simulink model "APB_Model0_v03_Test"  (R2020b)
settings: Solver=ode45  StartTime=0.0  StopTime=inf  RelTol=1e-3
undefined symbols (not defined in the file or in its folder): calb_Driver_acce, calb_Driver_bttn, calb_Driver_EmrBrk, calb_Driver_Prss, G_Fclamp, G_Kmot, G_Rmot, G_Stroke, G_SwOmega, GEN3, PbcDataStorageRequest_t
libraries: etargetslib x26, Lib_Op_Hndl x4, simulink x2, PbcOut_Checksum x2
(part 3 of 5)

== system APB_Model0_v03_Test/HstEcu/PBC/Subsystem/Subsystem3 ==
  PBCInMotorCurrentLeft_1ms : Inport
  Constant : Constant  Value=GEN3
  Delay : Delay  DelayLength=1
  Subsystem : Subsystem
  Subsystem4 : Subsystem
  Switch : Switch  Criteria=u2 ~= 0
  <phys_HwDrCt_ImotL> : Outport
  wires:
  Constant/1 -> Switch/2
  Subsystem4/1(Out1) -> Switch/1
  Subsystem/1(Out1) -> Switch/3
  Switch/1 -> <phys_HwDrCt_ImotL>/1
  PBCInMotorCurrentLeft_1ms/1 -> Delay/1
  Delay/1 -> Subsystem4/1(PBCInMotorCurrentLeft_1ms), Subsystem/1(PBCInMotorCurrentLeft_1ms)

== system APB_Model0_v03_Test/HstEcu/PBC/Subsystem/Subsystem4 ==
  PBCInMotorCurrentLeft_1ms : Inport
  Constant : Constant  Value=GEN3
  Delay : Delay  DelayLength=1
  Subsystem : Subsystem
  Subsystem4 : Subsystem
  Switch : Switch  Criteria=u2 ~= 0
  <phys_HwDrCt_ImotL> : Outport
  wires:
  PBCInMotorCurrentLeft_1ms/1 -> Delay/1
  Switch/1 -> <phys_HwDrCt_ImotL>/1
  Subsystem/1(Out1) -> Switch/3
  Subsystem4/1(Out1) -> Switch/1
  Constant/1 -> Switch/2
  Delay/1 -> Subsystem/1(PBCInMotorCurrentLeft_1ms), Subsystem4/1(PBCInMotorCurrentLeft_1ms)

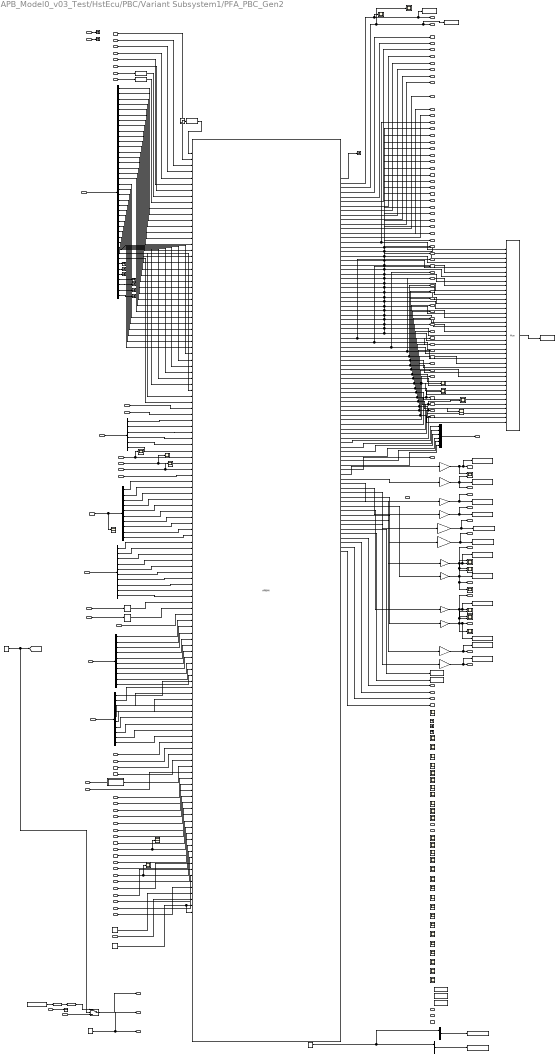
== system APB_Model0_v03_Test/HstEcu/PBC/Variant Subsystem1/PFA_PBC_Gen2 ==
  Pbc_Init : Inport
  Pbc_Cyclic : Inport  Port=2
  ApplyReleaseRequest : Inport  Port=3
  PBCInRollerBenchActive : Inport  Port=4
  PBCInLongAcceleration : Inport  Port=5
  PBCInMasterCylinderPressure : Inport  Port=6
  PBCInVehicleAmbientTemperature : Inport  Port=7
  PBCInWheelPressureFL : Inport  Port=8
  PBCInWheelPressureFR : Inport  Port=9
  PBCInWheelPressureRL : Inport  Port=10
  PBCInWheelPressureRR : Inport  Port=11
  PBCInWheelPressureReliabilityFL : Inport  Port=12
  PBCInWheelPressureReliabilityFR : Inport  Port=13
  PBCInWheelPressureReliabilityRL : Inport  Port=14
  PBCInWheelPressureReliabilityRR : Inport  Port=15
  PBCInWheelPulseFL : Inport  Port=16
  PBCInWheelPulseFR : Inport  Port=17
  PBCInWheelPulseRL : Inport  Port=18
  PBCInWheelPulseRR : Inport  Port=19
  PBCInWheelSPeedFL : Inport  Port=20
  PBCInWheelSPeedFR : Inport  Port=21
  PBCInWheelSPeedRL : Inport  Port=22
  PBCInWheelSPeedRR : Inport  Port=23
  PBCInDiagOperationMode : Inport  Port=24
  PBCInDiagRequest : Inport  Port=25
  PBCinHostSoftwareVersion : Inport  Port=26
  PBCInDataStorageValid1 : Inport  Port=27
  PBCInDataStorageValid2 : Inport  Port=28
  PBCInDataStorageValid3 : Inport  Port=29
  PBCInUnexpectedPowerDown : Inport  Port=30
  PBCInVariantItem : Inport  Port=31
  PBCInDataStorageRead1 : Inport  Port=32
  PBCInDataStorageRead9 : Inport  Port=33
  PBCInPbcSleepTime : Inport  Port=34
  PBCInFaultRecoveryRequest : Inport  Port=35
  PBCInHpsAvailability : Inport  Port=36
  PBCInHpsAcknowledge : Inport  Port=37
  PBCInMotorCurrentLeft_1ms : Inport  Port=38
  PBCInMotorCurrentRight_1ms : Inport  Port=39
  HWDriver_MotorVoltageLeft_1ms : Inport  Port=40
  HWDriver_MotorVoltageRight_1ms : Inport  Port=41
  PBCInMotorDriverSupplyVoltage : Inport  Port=42
  PBCinHostAvailabilityLeft : Inport  Port=43
  PBCinHostAvailabilityRight : Inport  Port=44
  PBCInMotorDriverStateLeft : Inport  Port=45
  PBCInMotorDriverStateRight : Inport  Port=46
  PBCInPowerSupplyState : Inport  Port=47
  PbcInMileage : Inport  Port=48
  PbcInEngineCranking : Inport  Port=49
  PbcInDriveAwayIntentionIndication : Inport  Port=50
  "PBCInDataStorageRead77 " : Inport  Port=51
  "PBCInDataStorage_Read " : Inport  Port=52
  OutOfSpec_Init : Inport  Port=53
  AcP00 : Scope
  AcP77 : Scope
  AcpData02 : Scope
  AcpData04 : Scope
  AssemblyChek : Scope
  Constant : Constant  Value=0
  Constant1 : Constant  Value=0
  Constant2 : Constant  Value=0  OutDataTypeStr=uint8
  Constant4 : Constant  Value=0
  Constant9 : Constant  Value=0  OutDataTypeStr=uint8
  Data Type Conversion{1,5,7..8} (4 alike) : DataTypeConversion  OutDataTypeStr=uint8
  Data Type Conversion6 : DataTypeConversion  OutDataTypeStr=boolean
  Data03 : Scope
  Data255 : Scope
  Demux1 : Demux  Outputs=40
  Demux{2..5} (4 alike) : Demux  Outputs=10
  Demux6 : Demux  Outputs=6
  EncodedAssembly : Scope
  From Workspace : FromWorkspace  VariableName=Memo1
  Gain{1,8,11..12} (4 alike) : Gain  Gain=G_Fclamp
  Gain10 : Gain  Gain=G_Rmot
  Gain2 : Gain  Gain=G_Stroke
  Gain3 : Gain  Gain=G_Stroke
  Gain4 : Gain  Gain=G_SwOmega
  Gain5 : Gain  Gain=G_SwOmega
  Gain6 : Gain  Gain=G_Kmot
  Gain7 : Gain  Gain=G_Kmot
  Gain9 : Gain  Gain=G_Rmot
  IsAllData : Scope
  IsAllDataInit : Scope
  IsIf1Reached : Scope
  IsIfaActive : Scope
  IsRelfinis : Scope  NumInputPorts=2
  Mux : Mux  Inputs=2
  Mux1 : Mux  Inputs=2
  Mux2 : Mux  Inputs=6
  Mux3 : Mux  Inputs=5
  Mux4 : Mux  Inputs=39
  Rate Transition42 : RateTransition  OutPortSampleTime=0.01
      settings: AttributesFormatString=%<OutPortSampleTime>
  Rate Transition43 : RateTransition  OutPortSampleTime=0.01
      settings: AttributesFormatString=%<OutPortSampleTime>
  ReleaseTim : Scope  NumInputPorts=2
  S-Function Builder1 : S-Function  InitFcn=try, set_param(gcb,'FunctionName','APBMi'), end  FunctionName=APBMi  SFunctionModules=APBMi_wrapper AcmBtmCalcStartBit AcmBtmCoolingAdjustmentConditions AcmBtmDTDiscCalcCooling AcmBtmDTDiscCalcHeating AcmBtmDTDiscSum AcmBtmFailureConditions AcmBtmInitStandstillCorrection AcmBtmMain AcmBtmOverheatCalc AcmBtmQualifierUpgrade AcmBtmSetFaultHandler AcmBtmSigPerm AcmBtmStatusCoding AcmBtmTambUpdate AcmBtmTDisc AcmBtmTrigger AcmBtmVelocityUpdate AcmBtmWheelXY AcpHemming AcpLibInCopy AcpLibOutCopy AcpLibWrapper AcpVariant ActuateReclamp ApplyPhaseStateMachine Ax2SlopeRaw a_intpol BtmInterfaceAdaption BtmTaskAdaption calcPbcActualMotorCommand calcPbcTargetMotorCommand CalcPostRunReq calcSwOmegaDot calcTargetStateDA Cal_VehicleSpeed ChangeTypeOfRC_HpsNotAcknowledged ChangeTypeOfRC_RDF_WithoutHps ChoiceOfCFS confEcuCodeGen_VDA_2 DataResetRequestDistinction Decoder_WSS_Quality DelayTimeCalculation DiagExecutionHandler DiagModeFConnectorOut DiagReqFeedback DiagRequestAccepter DiagRequestAckowledge_Enum_Map DiagRequestSplitter DiagRequest_Enum_Map DiagStateCalculation DiagStateHandler DSM_EmergencyReleaseSwitch DSM_FailureNode DSM_HostAvailabilityDecoder DSM_MainFailureHandler DSM_TargetStateIndependant DSM_TargetStateMain DSM_TargetStateMax dx_dt dx_dt0 EEPROM_Decoder_C EEPROM_Encoder_C EngineCranking ErrorRatioGoodCheckEncoder ForceEstimation HFBA_Repeater HostAvailabilityDetection HpsActivator HpsMerging HpsPressureChoice HpsSteering IfaTif_StateMachine InfoAchievedFClamp InfoAppCounter InfoBrakeTemperature InfoFLOne_TwoCounter InfoHPSRequestCounter InfoOutOfSpec InfoReclampCounter InfoReleaseCounter InitialConditionsforRWU InitStateCalculation isEndOfIdlePhase isForceEstimationActivate isMotParValid isRwuExecutionPossible isSwitchOnPeakPresent isTDiscRearMaxValid LateEngineCranking LockReleaseExecutionHandler LockReleaseStatemachine MileageSinceLastParkApplied MileageValidity MocOff_DeltaF_Addition MonIDs MON_ActuatorModeInitMonitoring MON_ActuatorModeOperationMonitoring MON_DegradationManager MON_DevEncoder MON_DevEncoderInit_APBDi MON_DiagnosisDetector MON_DynLockDetector MON_EmergencyReleaseDetectionDurRel MON_EngineCranking MON_ErrorRatioGoodCheckEncoder MON_GradientMonitoringForceBuildUpDurLock MON_HPSRequestFailureDurLock MON_IdleSpindleStrokeMonitoringDurLock MON_IdleTorqueMonitoringDurLock MON_MotorControlDetectionDurAppl MON_MotorParameterMonitoringDurLock MON_TimeoutMonitoringForceBuildUpDurLock NoActuation OngoingActuation OnGoingActuationExtended OutOfSpec PAAMerging PadAdjustmentRequest ParAcp_BrakeDiscTemperatureModel ParAcp_BTM_Calibration ParAcp_BTM_FA ParAcp_BTM_RA ParAcp_Constant ParAcp_DynamicStateManager ParAcp_HpsDevice ParAcp_HWDriver ParAcp_InfoService ParAcp_Monitoring ParAcp_MotorControl ParAcp_PadAdjust ParAcp_RecalibrationFunction ParAcp_RollDetection ParAcp_RWU ParAcp_SlopeCalculation ParAcp_TargetActuation ParkBrakeControl_T10ms_VDA_2 ParkBrakeControl_VDA_2 PbcBTM PbcBTM_PdmValueValidAdaption PbcChronometre PbcCtrlBothWheels PbcCtrlOneWheel PbcDynamicStateManager PbcForceEstimation PbcHpsChronometre PbcHpsDevice PbcHWDriverCommand PbcHWDriverCommandBothWheels PbcIfPDM PbcInfoService PbcMotorControl PbcMovementDetection PbcPadAdjustment PbcQDotReader PbcQDotReaderSoPeak PbcRecalibrationFunction PbcRoadSlope_availability PbcRollDetection PbcRWU PbcRwuSlip PbcSignalConditioning PbcSlopeCalculation PbcSpeedCalculation PbcTargetActuation PbcVehicleMovementDetection PbcWheelMovementDetection PBC_BoschCbi_VDA_2 Pbc_dcTLA Pbc_dcTLA_ClampingForceTable Pbc_DcTLA_StateMachine Pbc_FClampTarBySlope_CBI Pbc_ParkBrakeSupportRequest Pbc_prepressure_calculation Pbc_Pressure4StandstillDetection_CBI Pbc_ReclampType_Merging Pbc_VDAtwo Pbc_VHC PdmActuatorState PdmBtm PdmDataValid PTAMerging RecalibrationTrigger RecogTouchPoints RollAwayValidation RollerBenchHandler RWU_StateMachine SIC_APBMi SIC_Calc_R_K_Mot SIC_IdlePhaseParameter SIC_InrushPeakDetector SIC_MotorCurrent SIC_MotorCurrentConcentrator SIC_MotorCurrentCtrl SIC_MotorParameter SIC_MotorResidualCurrent SIC_MotorVoltage SIC_PistonStroke Signal_Availability_sint Signal_Availability_sint0 Signal_Availability_sint1 Signal_Availability_uint Signal_Availability_uint0 Signal_Availability_uint1 StateRequestCalculation StopImmediatelyCalculation StopImmediatelyCalculationLR TargetStateRDF TestCalc0xFF TestValue_C WheelPressureReliability_Enum_Map _BTM_Constant _Environment_QualityGrades MON_APBMi ActuateAllReleases ActuateByForce ActuatorStateMerging ApplyReleaseMerging CFS_IndependentActuation DevelopmentMessagesEncoding DevelpmentMessagesPreparation DiagModeFConnector DoubleApplyFunction DSM_FaultStatusMerging EEPROM_Boolean_Coder ForceEstimationVoltTempFactor HpsRequestMerging IndependantActuationConfig InfoOutOfSpecBlock isActuatorFinalState LongAccelerationManagement MergeParkBrakeSupportRequest MON_AbutmentDetectionDurRel MON_DisableMonitoring MON_ForcedGoodCheck MON_FreeLoadDetectionDurRel MON_HostDown MON_InfoFaultMonitoring MON_LeftRightIncoherence MON_MotorStartDetection MON_Overvoltage MON_SideSelfIncoherence MON_SuspicousReleasedDetector MON_Undervoltage OosActivator OosAxInvalid OosCbiStar OosDataStorage3Invalid OosIndependentControl OosMerger OosSlopeInvalid ParAcp_ForceEstimation ParAcp_InputHandling ParAcp_SignalConditioning Pbc_FClamp_PostRunTimeTgt Pbc_hRCWithoutHps Pbc_TemperatureSlopePressure_SliceChoice PbcDevelopmentMessages PbcForceEstimationOp PbcInputHandler PbcPistonPositionEstimation PbcVariantConfig PdmRollAway RequestProcesser TestCalcInit WaitRecoveryActuationEnded HostAvailabilityMerging Pbc_ReleaseStroke_Calculation VoltageVariationDetection  SFunctionDeploymentMode=off  EnableBusSupport=off  mask(S-Function Builder){}
      mask help: The S-Function Builder block creates a wrapper C-MEX S-function from your supplied C code with multiple input ports, output ports, and a variable number of scalar, vector, or matrix parameters. The input and output ports can propagate Simulink built-in data types, fixed-point datatypes, complex, frame, 1-D, and 2-D signals. This block also supports discrete and continuous states of type real. You can optionally have the block generate a TLC file to be used with Real-Time Workshop for code generation.
      mask init:
      | val = [[.9  0.75 0.75 1 1 .9 .9 1]',[1 1 0.75 0.75 .9 .9 1 .9]'];try , sys = get_param(gcb,'SfunBuilderFcnName');if isempty(sys), sys = get_param(gcb,'FunctionName'); end,catch, sys = get_param(gcb,'FunctionName'); end
      settings: AttributesFormatString=%<SFunctionModules>\n%<FunctionName>  CopyFcn=set_param(gcbh,'LinkStatus','none')  PreSaveFcn=try, set_param(gcb,'FunctionName','APBMi'), end  OpenFcn=sfunctionwizard(gcbh)
      mask Display: plot(val(:,1),val(:,2)),disp(sys),port_label('input',1,'triggerInFirstCall'),port_label('input',2,'PBCInApplyReleaseRequest'),port_label('input',3,'PBCInDataStorageRead1'),port_label('input',4,'PBCInDataStorageRead9'),port_label('input',5,'PBCInDataStorageValid1'),port_label('input',6,'PBCInDataStorageValid2'),port_label('input',7,'PBCInDataStorageValid3'),port_label('input',8,'PBCInDiagOperationMode'),port_label('input',9,'PBCInDiagRequest'),port_label('input',10,'PBCInFaultRecoveryRequest_01'),port_label('input',11,'PBCInFaultRecoveryRequest_02'),port_label('input',12,'PBCInFaultRecoveryRequest_03'),port_label('input',13,'PBCInFaultRecoveryRequest_04'),port_label('input',14,'PBCInFaultRecoveryRequest_05'),port_label('input',15,'PBCInFaultRecoveryRequest_06'),port_label('input',16,'PBCInFaultRecoveryRequest_07'),port_label('input',17,'PBCInFaultRecoveryRequest_08'),port_label('input',18,'PBCInFaultRecoveryRequest_09'),port_label('input',19,'PBCInFaultRecoveryRequest_10'),port_label('input',20,'PBCInFaultRecoveryRequest_11'),port_label('input',21,'PBCInFaultRecoveryRequest_12'),port_label('input',22,'PBCInFaultRecoveryRequest_13'),port_label('input',23,'PBCInFaultRecoveryRequest_14'),port_label('input',24,'PBCInFaultRecoveryRequest_15'),port_label('input',25,'PBCInFaultRecoveryRequest_16'),port_label('input',26,'PBCInFaultRecoveryRequest_17'),port_label('input',27,'PBCInFaultRecoveryRequest_18'),port_label('input',28,'PBCInFaultRecoveryRequest_19'),port_label('input',29,'PBCInFaultRecoveryRequest_20'),port_label('input',30,'PBCInFaultRecoveryRequest_21'),port_label('input',31,'PBCInFaultRecoveryRequest_22'),port_label('input',32,'PBCInFaultRecoveryRequest_23'),port_label('input',33,'PBCInFaultRecoveryRequest_24'),port_label('input',34,'PBCInFaultRecoveryRequest_25'),port_label('input',35,'PBCInFaultRecoveryRequest_26'),port_label('input',36,'PBCInFaultRecoveryRequest_27'),port_label('input',37,'PBCInFaultRecoveryRequest_29'),port_label('input',38,'PBCInFaultRecoveryRequest_30'),port_label('input',39,'PBCInFaultRecoveryRequest_31'),port_label('input',40,'PBCInFaultRecoveryRequest_32'),port_label('input',41,'PBCInFaultRecoveryRequest_33'),port_label('input',42,'PBCInFaultRecoveryRequest_39'),port_label('input',43,'PBCInHostAvailabilityLeft'),port_label('input',44,'PBCInHostAvailabilityRight'),port_label('input',45,'PBCInHostSoftwareVersion0'),port_label('input',46,'PBCInHostSoftwareVersion1'),port_label('input',47,'PBCInHostSoftwareVersion2'),port_label('input',48,'PBCInHostSoftwareVersion3'),port_label('input',49,'PBCInHostSoftwareVersion4'),port_label('input',50,'PBCInHostSoftwareVersion5'),port_label('input',51,'PBCInHpsAvailability'),port_label('input',52,'PBCInHpsAcknowledge'),port_label('input',53,'PBCInLongAcceleration'),port_label('input',54,'PBCInMasterCylinderPressure'),port_label('input',55,'PBCInMotorCurrentLeft_K0'),port_label('input',56,'PBCInMotorCurrentLeft_K1'),port_label('input',57,'PBCInMotorCurrentLeft_K2'),port_label('input',58,'PBCInMotorCurrentLeft_K3'),port_label('input',59,'PBCInMotorCurrentLeft_K4'),port_label('input',60,'PBCInMotorCurrentLeft_K5'),port_label('input',61,'PBCInMotorCurrentLeft_K6'),port_label('input',62,'PBCInMotorCurrentLeft_K7'),port_label('input',63,'PBCInMotorCurrentLeft_K8'),port_label('input',64,'PBCInMotorCurrentLeft_K9'),port_label('input',65,'PBCInMotorCurrentRight_K0'),port_label('input',66,'PBCInMotorCurrentRight_K1'),port_label('input',67,'PBCInMotorCurrentRight_K2'),port_label('input',68,'PBCInMotorCurrentRight_K3'),port_label('input',69,'PBCInMotorCurrentRight_K4'),port_label('input',70,'PBCInMotorCurrentRight_K5'),port_label('input',71,'PBCInMotorCurrentRight_K6'),port_label('input',72,'PBCInMotorCurrentRight_K7'),port_label('input',73,'PBCInMotorCurrentRight_K8'),port_label('input',74,'PBCInMotorCurrentRight_K9'),port_label('input',75,'PBCInMotorDriverStateLeft'),port_label('input',76,'PBCInMotorDriverStateRight'),port_label('input',77,'PBCInMotorDriverSupplyVoltage'),port_label('input',78,'PBCInMotorVoltageLeft_K0'),port_label('input',79,'PBCInMotorVoltageLeft_K1'),port_label('input',80,'PBCInMotorVoltageLeft_K2'),port_label('input',81,'PBCInMotorVoltageLeft_K3'),port_label('input',82,'PBCInMotorVoltageLeft_K4'),port_label('input',83,'PBCInMotorVoltageLeft_K5'),port_label('input',84,'PBCInMotorVoltageLeft_K6'),port_label('input',85,'PBCInMotorVoltageLeft_K7'),port_label('input',86,'PBCInMotorVoltageLeft_K8'),port_label('input',87,'PBCInMotorVoltageLeft_K9'),port_label('input',88,'PBCInMotorVoltageRight_K0'),port_label('input',89,'PBCInMotorVoltageRight_K1'),port_label('input',90,'PBCInMotorVoltageRight_K2'),port_label('input',91,'PBCInMotorVoltageRight_K3'),port_label('input',92,'PBCInMotorVoltageRight_K4'),port_label('input',93,'PBCInMotorVoltageRight_K5'),port_label('input',94,'PBCInMotorVoltageRight_K6'),port_label('input',95,'PBCInMotorVoltageRight_K7'),port_label('input',96,'PBCInMotorVoltageRight_K8'),port_label('input',97,'PBCInMotorVoltageRight_K9'),port_label('input',98,'PBCInPowerSupplyState'),port_label('input',99,'PBCInRollerBenchActive'),port_label('input',100,'PBCInPbcSleepTime'),port_label('input',101,'PBCInUnexpectedPowerDown'),port_label('input',102,'PBCInVariantItem'),port_label('input',103,'PBCInVehicleAmbientTemperature'),port_label('input',104,'PBCInWheelPressureFrontLeft'),port_label('input',105,'PBCInWheelPressureFrontRight'),port_label('input',106,'PBCInWheelPressureRearLeft'),port_label('input',107,'PBCInWheelPressureRearRight'),port_label('input',108,'PBCInWheelPressureReliabilityFrontLeft'),port_label('input',109,'PBCInWheelPressureReliabilityFrontRight'),port_label('input',110,'PBCInWheelPressureReliabilityRearLeft'),port_label('input',111,'PBCInWheelPressureReliabilityRearRight'),port_label('input',112,'PBCInWheelPulseFrontLeft'),port_label('input',113,'PBCInWheelPulseFrontRight'),port_label('input',114,'PBCInWheelPulseRearLeft'),port_label('input',115,'PBCInWheelPulseRearRight'),port_label('input',116,'PBCInWheelSpeedFrontLeft'),port_label('input',117,'PBCInWheelSpeedFrontRight'),port_label('input',118,'PBCInWheelSpeedRearLeft'),port_label('input',119,'PBCInWheelSpeedRearRight'),port_label('input',120,'PbcInEngineCranking'),port_label('input',121,'PbcInMileage'),port_label('input',122,'PbcInDriveAwayIntentionIndication'),port_label('input',123,'PBCInDataStorageRead105'),port_label('input',124,'PBCInDataStorageRead77'),port_label('input',125,'PBCInDataStorageRead80'),port_label('input',126,'PBCInDataStorageRead91'),port_label('input',127,'PBCInDataStorageRead92'),port_label('input',128,'PBCInDataStorageRead93'),port_label('input',129,'PBCInDataStorageRead94'),port_label('input',130,'PBCInDataStorageRead95'),port_label('input',131,'PBCInDataStorageRead96'),port_label('input',132,'PBCInDataStorageRead97'),port_label('input',133,'PBCInDataStorageRead2'),port_label('input',134,'PBCInDataStorageRead3'),port_label('input',135,'PBCInDataStorageRead10'),port_label('input',136,'PBCInDataStorageRead142'),port_label('input',137,'MDbgFClampTar'),port_label('input',138,'MDbg_factorV_Left_F1'),port_label('input',139,'MDbg_factorT_Left_F1'),port_label('input',140,'MDbg_factorV_Left_F2'),port_label('input',141,'MDbg_factorT_Left_F2'),port_label('input',142,'MDbg_factorV_Right_F1'),port_label('input',143,'MDbg_factorT_Right_F1'),port_label('input',144,'MDbg_factorV_Right_F2'),port_label('input',145,'MDbg_factorT_Right_F2'),port_label('output',1,'triggerOutFirstCall'),port_label('output',2,'PBCOutActuatorStateLeft'),port_label('output',3,'PBCOutActuatorStateRight'),port_label('output',4,'PBCOutDataStorageWrite1'),port_label('output',5,'PBCOutDataStorageWrite9'),port_label('output',6,'PBCOutDevelopmentMessages0'),port_label('output',7,'PBCOutDiagAchievedClampingForceLeft'),port_label('output',8,'PBCOutDiagAchievedClampingForceRight'),port_label('output',9,'PBCOutDiagActuationCounterLeft'),port_label('output',10,'PBCOutDiagActuationCounterRight'),port_label('output',11,'PBCOutDiagBrakeTemperatureLeft'),port_label('output',12,'PBCOutDiagBrakeTemperatureRight'),port_label('output',13,'PBCOutDiagRequestAcknowledge'),port_label('output',14,'PBCOutDiagRequestStatus'),port_label('output',15,'PBCOutFaultStatus_01'),port_label('output',16,'PBCOutFaultStatus_02'),port_label('output',17,'PBCOutFaultStatus_03'),port_label('output',18,'PBCOutFaultStatus_04'),port_label('output',19,'PBCOutFaultStatus_05'),port_label('output',20,'PBCOutFaultStatus_06'),port_label('output',21,'PBCOutFaultStatus_07'),port_label('output',22,'PBCOutFaultStatus_08'),port_label('output',23,'PBCOutFaultStatus_09'),port_label('output',24,'PBCOutFaultStatus_10'),port_label('output',25,'PBCOutFaultStatus_11'),port_label('output',26,'PBCOutFaultStatus_12'),port_label('output',27,'PBCOutFaultStatus_13'),port_label('output',28,'PBCOutFaultStatus_14'),port_label('output',29,'PBCOutFaultStatus_15'),port_label('output',30,'PBCOutFaultStatus_16'),port_label('output',31,'PBCOutFaultStatus_17'),port_label('output',32,'PBCOutFaultStatus_18'),port_label('output',33,'PBCOutFaultStatus_19'),port_label('output',34,'PBCOutFaultStatus_20'),port_label('output',35,'PBCOutFaultStatus_21'),port_label('output',36,'PBCOutFaultStatus_22'),port_label('output',37,'PBCOutFaultStatus_23'),port_label('output',38,'PBCOutFaultStatus_24'),port_label('output',39,'PBCOutFaultStatus_25'),port_label('output',40,'PBCOutFaultStatus_26'),port_label('output',41,'PBCOutFaultStatus_27'),port_label('output',42,'PBCOutFaultStatus_28'),port_label('output',43,'PBCOutFaultStatus_29'),port_label('output',44,'PBCOutFaultStatus_30'),port_label('output',45,'PBCOutFaultStatus_31'),port_label('output',46,'PBCOutFaultStatus_32'),port_label('output',47,'PBCOutFaultStatus_33'),port_label('output',48,'PBCOutFaultStatus_34'),port_label('output',49,'PBCOutFaultStatus_35'),port_label('output',50,'PBCOutFaultStatus_36'),port_label('output',51,'PBCOutFaultStatus_37'),port_label('output',52,'PBCOutFaultStatus_38'),port_label('output',53,'PBCOutFaultStatus_39'),port_label('output',54,'PBCOutHpsPressure'),port_label('output',55,'PBCOutHpsRequest'),port_label('output',56,'PBCOutMotorCommandLeft'),port_label('output',57,'PBCOutMotorCommandRight'),port_label('output',58,'PBCOutOutOfSpecMsg'),port_label('output',59,'PBCOutPbcSoftwareVersion0'),port_label('output',60,'PBCOutPbcSoftwareVersion1'),port_label('output',61,'PBCOutPbcSoftwareVersion2'),port_label('output',62,'PBCOutPbcSoftwareVersion3'),port_label('output',63,'PBCOutPbcSoftwareVersion4'),port_label('output',64,'PBCOutPbcSoftwareVersion5'),port_label('output',65,'PBCOutEcuPowerLatchRequest'),port_label('output',66,'PBCinternalFclampR'),port_label('output',67,'PBCinternalFclampL'),port_label('output',68,'PBCinternalSwStrokeR'),port_label('output',69,'PBCinternalSwStrokeL'),port_label('output',70,'PBCinternalSwOmegaR'),port_label('output',71,'PBCinternalSwOmegaL'),port_label('output',72,'PBCinternalKMotR'),port_label('output',73,'PBCinternalKMotL'),port_label('output',74,'PBCinternalRMotR'),port_label('output',75,'PBCinternalRMotL'),port_label('output',76,'PBCinternalFtarR'),port_label('output',77,'PBCinternalFtarL'),port_label('output',78,'PBCinternalTargetActuationR'),port_label('output',79,'PBCinternalTargetActuationL'),port_label('output',80,'PbcOutPadAdjustmentRequest'),port_label('output',81,'PbcOutParkSupportRequest'),port_label('output',82,'PbcOutDataStorageRequest'),port_label('output',83,'TriggerRecalibration'),port_label('output',84,'FachivedL'),port_label('output',85,'FachivedR'),port_label('output',86,'apprealreq'),port_label('output',87,'Motorcurrent'),port_label('output',88,'Motorvoltage'),port_label('output',89,'version4'),port_label('output',90,'version3'),port_label('output',91,'version2'),port_label('output',92,'version1'),port_label('output',93,'version0'),port_label('output',94,'MApplyReleaseRequestin'),port_label('output',95,'MTargetStateMainL'),port_label('output',96,'MTargetStateMainR'),port_label('output',97,'MUMotFLeft'),port_label('output',98,'MIMotFLeft'),port_label('output',99,'MIMotByForceLeft'),port_label('output',100,'MIMotResLeft'),port_label('output',101,'MIMotGradLeft'),port_label('output',102,'MIMotIdleLeft'),port_label('output',103,'MIMotIdleSeqLeft'),port_label('output',104,'MUMotIdleLeft'),port_label('output',105,'MKMotLeft'),port_label('output',106,'MRMotLeft'),port_label('output',107,'MMotParamQualifierLeft'),port_label('output',108,'MPistonStrokeLeft'),port_label('output',109,'MPistonStrokeFreeLoadLeft'),port_label('output',110,'MPistonStrokeFreeLoadT1Left'),port_label('output',111,'MPistonStrokeFreeLoadT2Left'),port_label('output',112,'MPistonStrokeT1Left'),port_label('output',113,'MPistonStrokeT2Left'),port_label('output',114,'MwMotFLeft'),port_label('output',115,'MPbcApplyPhaseLeft'),port_label('output',116,'MFEstLeft'),port_label('output',117,'MMInertiaLeft'),port_label('output',118,'MDeltaF_FEstLeft'),port_label('output',119,'MFEst_incl_MoCOffLeft'),port_label('output',120,'MFEstoptimalVTLeft'),port_label('output',121,'MisOuterAbutmentTouchedLeft'),port_label('output',122,'MisTouchPointReachedLeft'),port_label('output',123,'MPbcTargetMotorCommandLeft'),port_label('output',124,'MisActuationFinishedLeft'),port_label('output',125,'MisOptReleaseTimeReachedLeft'),port_label('output',126,'MisReleaseStrokeReachedLeft'),port_label('output',127,'MisReleaseTimeReachedLeft'),port_label('output',128,'MisReleasingIFAOverLeft'),port_label('output',129,'MisLockingFinishedLeft'),port_label('output',130,'MUMotFRight'),port_label('output',131,'MIMotFRight'),port_label('output',132,'MIMotByForceRight'),port_label('output',133,'MIMotResRight'),port_label('output',134,'MIMotGradRight'),port_label('output',135,'MIMotIdleRight'),port_label('output',136,'MIMotIdleSeqRight'),port_label('output',137,'MUMotIdleRight'),port_label('output',138,'MKMotRight'),port_label('output',139,'MRMotRight'),port_label('output',140,'MMotParamQualifierRight'),port_label('output',141,'MPistonStrokeRight'),port_label('output',142,'MPistonStrokeFreeLoadRight'),port_label('output',143,'MPistonStrokeFreeLoadT1Right'),port_label('output',144,'MPistonStrokeFreeLoadT2Right'),port_label('output',145,'MPistonStrokeT1Right'),port_label('output',146,'MPistonStrokeT2Right'),port_label('output',147,'MwMotFRight'),port_label('output',148,'MPbcApplyPhaseRight'),port_label('output',149,'MFEstRight'),port_label('output',150,'MMInertiaRight'),port_label('output',151,'MDeltaF_FEstRight'),port_label('output',152,'MFEst_incl_MoCOffRight'),port_label('output',153,'MFEstoptimalVTRight'),port_label('output',154,'MisOuterAbutmentTouchedRight'),port_label('output',155,'MisTouchPointReachedRight'),port_label('output',156,'MPbcTargetMotorCommandRight'),port_label('output',157,'MisActuationFinishedRight'),port_label('output',158,'MisOptReleaseTimeReachedRight'),port_label('output',159,'MisReleaseStrokeReachedRight'),port_label('output',160,'MisReleaseTimeReachedRight'),port_label('output',161,'MisReleasingIFAOverRight'),port_label('output',162,'MisLockingFinishedRight'),port_label('output',163,'MIMotMeasLeft'),port_label('output',164,'MIMotMeasRight'),port_label('output',165,'MIMotF_L'),port_label('output',166,'MIMotF_R'),port_label('output',167,'MKMot_L'),port_label('output',168,'MKMot_R'),port_label('output',169,'MRMot_L'),port_label('output',170,'MRMot_R'),port_label('output',171,'MFEstoptimalVT_L'),port_label('output',172,'MFEstoptimalVT_R'),port_label('output',173,'MPistonStroke_L'),port_label('output',174,'MPistonStroke_R'),port_label('output',175,'MPistonStrokeFL_L'),port_label('output',176,'MPistonStrokeFL_R'),port_label('output',177,'MwMotF_L'),port_label('output',178,'MwMotF_R'),port_label('output',179,'AcpOutMotorCommandL'),port_label('output',180,'AcpOutMotorCommandR'),port_label('output',181,'AcpInMotorDriverStateL'),port_label('output',182,'AcpInMotorDriverStateR')
  Scope{,1..5,7,9,12..14,16..19,22..25,27..28} (21 alike) : Scope
  Scope{6,8,10..11,15,21,26} (7 alike) : Scope  NumInputPorts=2
  Scope20 : Scope  NumInputPorts=3
  Step : Step  Time=0.02  Before=1  After=0
  Subsystem : Subsystem
  Switch : Switch  Criteria=u2 ~= 0
  TargetstateMain : Scope  NumInputPorts=2
  Terminator{,1..13} (14 alike) : Terminator
  To Workspace : ToWorkspace  VariableName=Faulty  SaveFormat=Timeseries  SampleTime=-1
  To Workspace1 : ToWorkspace  VariableName=FclampLeft1  SampleTime=-1
  To Workspace10 : ToWorkspace  VariableName=RMotRight1  SampleTime=-1
  To Workspace11 : ToWorkspace  VariableName=FTarR1  SampleTime=-1
  To Workspace12 : ToWorkspace  VariableName=FTarL1  SampleTime=-1
  To Workspace13 : ToWorkspace  VariableName=TargetActuationR1  SampleTime=-1
  To Workspace14 : ToWorkspace  VariableName=TargetActuationL1  SampleTime=-1
  To Workspace15 : ToWorkspace  VariableName=TDiscMax1  SaveFormat=Timeseries  SampleTime=-1
  To Workspace16 : ToWorkspace  VariableName=TDiscRL1  SaveFormat=Timeseries  SampleTime=-1
  To Workspace17 : ToWorkspace  VariableName=TDiscRR1  SaveFormat=Timeseries  SampleTime=-1
  To Workspace18 : ToWorkspace  VariableName=PBCSL  SaveFormat=Timeseries  SampleTime=-1
  To Workspace19 : ToWorkspace  VariableName=PBCSR  SaveFormat=Timeseries  SampleTime=-1
  To Workspace2 : ToWorkspace  VariableName=FclampRight1  SampleTime=-1
  To Workspace20 : ToWorkspace  VariableName=PBCOutDataStorageWrite  SaveFormat=Timeseries  SampleTime=-1
  To Workspace21 : ToWorkspace  VariableName=PBCOutDataStorageWrite1  SaveFormat=Timeseries  SampleTime=-1
  To Workspace3 : ToWorkspace  VariableName=StrokeLeft1  SampleTime=-1
  To Workspace4 : ToWorkspace  VariableName=StrokeRight1  SampleTime=-1
  To Workspace5 : ToWorkspace  VariableName=SwOmegaLeft1  SampleTime=-1
  To Workspace6 : ToWorkspace  VariableName=SwOmegaRight1  SampleTime=-1
  To Workspace7 : ToWorkspace  VariableName=KMotRight1  SampleTime=-1
  To Workspace8 : ToWorkspace  VariableName=KMotLeft1  SampleTime=-1
  To Workspace9 : ToWorkspace  VariableName=RMotLeft1  SampleTime=-1
  cnt : Scope
  right : Scope  NumInputPorts=2
  slip : Scope
  triggerRecalibration : Scope
  PBCOutActuatorStateLeft : Outport  VectorParamsAs1DForOutWhenUnconnected=off
  PBCOutActuatorStateRight : Outport  Port=2  VectorParamsAs1DForOutWhenUnconnected=off
  PBCOutDataStorageWrite1 : Outport  Port=3  VectorParamsAs1DForOutWhenUnconnected=off
  PBCOutDataStorageWrite9 : Outport  Port=4  VectorParamsAs1DForOutWhenUnconnected=off
  PBCOutDevelopmentMessages0 : Outport  Port=5  VectorParamsAs1DForOutWhenUnconnected=off
  PBCOutDiagAchievedClampingForceLeft : Outport  Port=6  VectorParamsAs1DForOutWhenUnconnected=off
  PBCOutDiagAchievedClampingForceRight : Outport  Port=7  VectorParamsAs1DForOutWhenUnconnected=off
  PBCOutDiagActuationCounterLeft : Outport  Port=8  VectorParamsAs1DForOutWhenUnconnected=off
  PBCOutDiagActuationCounterRight : Outport  Port=9  VectorParamsAs1DForOutWhenUnconnected=off
  PBCOutDiagBrakeTemperatureLeft : Outport  Port=10  VectorParamsAs1DForOutWhenUnconnected=off
  PBCOutDiagBrakeTemperatureRight : Outport  Port=11  VectorParamsAs1DForOutWhenUnconnected=off
  PBCOutDiagRequestAcknowledge : Outport  Port=12  VectorParamsAs1DForOutWhenUnconnected=off
  PBCOutDiagRequestStatus : Outport  Port=13  VectorParamsAs1DForOutWhenUnconnected=off
  PBCOutFaultStatus_01 : Outport  Port=14  VectorParamsAs1DForOutWhenUnconnected=off
  PBCOutFaultStatus_02 : Outport  Port=15  VectorParamsAs1DForOutWhenUnconnected=off
  PBCOutFaultStatus_03 : Outport  Port=16  VectorParamsAs1DForOutWhenUnconnected=off
  PBCOutFaultStatus_04 : Outport  Port=17  VectorParamsAs1DForOutWhenUnconnected=off
  PBCOutFaultStatus_05 : Outport  Port=18  VectorParamsAs1DForOutWhenUnconnected=off
  PBCOutFaultStatus_06 : Outport  Port=19  VectorParamsAs1DForOutWhenUnconnected=off
  PBCOutFaultStatus_07 : Outport  Port=20  VectorParamsAs1DForOutWhenUnconnected=off
  PBCOutFaultStatus_08 : Outport  Port=21  VectorParamsAs1DForOutWhenUnconnected=off
  PBCOutFaultStatus_09 : Outport  Port=22  VectorParamsAs1DForOutWhenUnconnected=off
  PBCOutFaultStatus_10 : Outport  Port=23  VectorParamsAs1DForOutWhenUnconnected=off
  PBCOutFaultStatus_11 : Outport  Port=24  VectorParamsAs1DForOutWhenUnconnected=off
  PBCOutFaultStatus_12 : Outport  Port=25  VectorParamsAs1DForOutWhenUnconnected=off
  PBCOutFaultStatus_13 : Outport  Port=26  VectorParamsAs1DForOutWhenUnconnected=off
  PBCOutFaultStatus_14 : Outport  Port=27  VectorParamsAs1DForOutWhenUnconnected=off
  PBCOutFaultStatus_15 : Outport  Port=28  VectorParamsAs1DForOutWhenUnconnected=off
  PBCOutFaultStatus_16 : Outport  Port=29  VectorParamsAs1DForOutWhenUnconnected=off
  PBCOutFaultStatus_17 : Outport  Port=30  VectorParamsAs1DForOutWhenUnconnected=off
  PBCOutFaultStatus_18 : Outport  Port=31  VectorParamsAs1DForOutWhenUnconnected=off
  PBCOutFaultStatus_19 : Outport  Port=32  VectorParamsAs1DForOutWhenUnconnected=off
  PBCOutFaultStatus_20 : Outport  Port=33  VectorParamsAs1DForOutWhenUnconnected=off
  PBCOutFaultStatus_21 : Outport  Port=34  VectorParamsAs1DForOutWhenUnconnected=off
  PBCOutFaultStatus_22 : Outport  Port=35  VectorParamsAs1DForOutWhenUnconnected=off
  PBCOutFaultStatus_23 : Outport  Port=36  VectorParamsAs1DForOutWhenUnconnected=off
  PBCOutFaultStatus_24 : Outport  Port=37  VectorParamsAs1DForOutWhenUnconnected=off
  PBCOutFaultStatus_25 : Outport  Port=38  VectorParamsAs1DForOutWhenUnconnected=off
  PBCOutFaultStatus_26 : Outport  Port=39  VectorParamsAs1DForOutWhenUnconnected=off
  PBCOutFaultStatus_27 : Outport  Port=40  VectorParamsAs1DForOutWhenUnconnected=off
  PBCOutFaultStatus_28 : Outport  Port=41  VectorParamsAs1DForOutWhenUnconnected=off
  PBCOutFaultStatus_29 : Outport  Port=42  VectorParamsAs1DForOutWhenUnconnected=off
  PBCOutFaultStatus_30 : Outport  Port=43  VectorParamsAs1DForOutWhenUnconnected=off
  PBCOutFaultStatus_31 : Outport  Port=44  VectorParamsAs1DForOutWhenUnconnected=off
  PBCOutFaultStatus_32 : Outport  Port=45  VectorParamsAs1DForOutWhenUnconnected=off
  PBCOutFaultStatus_33 : Outport  Port=46  VectorParamsAs1DForOutWhenUnconnected=off
  PBCOutFaultStatus_34 : Outport  Port=47  VectorParamsAs1DForOutWhenUnconnected=off
  PBCOutFaultStatus_35 : Outport  Port=48  VectorParamsAs1DForOutWhenUnconnected=off
  PBCOutFaultStatus_36 : Outport  Port=49  VectorParamsAs1DForOutWhenUnconnected=off
  PBCOutFaultStatus_37 : Outport  Port=50  VectorParamsAs1DForOutWhenUnconnected=off
  PBCOutFaultStatus_38 : Outport  Port=51  VectorParamsAs1DForOutWhenUnconnected=off
  PBCOutFaultStatus_39 : Outport  Port=52  VectorParamsAs1DForOutWhenUnconnected=off
  PBCOutHpsPressure : Outport  Port=53  VectorParamsAs1DForOutWhenUnconnected=off
  PBCOutHpsRequest : Outport  Port=54  VectorParamsAs1DForOutWhenUnconnected=off
  PBCOutMotorCommandLeft : Outport  Port=55  VectorParamsAs1DForOutWhenUnconnected=off
  PBCOutMotorCommandRight : Outport  Port=56  VectorParamsAs1DForOutWhenUnconnected=off
  PBCOutOfSpecMsg : Outport  Port=57  VectorParamsAs1DForOutWhenUnconnected=off
  PBCOutEcuPowerLatchRequest : Outport  Port=58  VectorParamsAs1DForOutWhenUnconnected=off
  F_clamp : Outport  Port=59  VectorParamsAs1DForOutWhenUnconnected=off
  PbcOutPadAdjustmentRequest : Outport  Port=60  VectorParamsAs1DForOutWhenUnconnected=off
  "PbcOutDataStorageRequest " : Outport  Port=61  VectorParamsAs1DForOutWhenUnconnected=off
  PbcOutParkSupportRequest : Outport  Port=62  VectorParamsAs1DForOutWhenUnconnected=off
  triggerrecal : Outport  Port=63  VectorParamsAs1DForOutWhenUnconnected=off
  FclampRight : Outport  Port=64  VectorParamsAs1DForOutWhenUnconnected=off
  FclampLeft : Outport  Port=65  VectorParamsAs1DForOutWhenUnconnected=off
  StrokeRight : Outport  Port=66  VectorParamsAs1DForOutWhenUnconnected=off
  StrokeLeft : Outport  Port=67  VectorParamsAs1DForOutWhenUnconnected=off
  SwOmegaRight : Outport  Port=68  VectorParamsAs1DForOutWhenUnconnected=off
  SwOmegaLeft : Outport  Port=69  VectorParamsAs1DForOutWhenUnconnected=off
  KMotLeft : Outport  Port=70  VectorParamsAs1DForOutWhenUnconnected=off
  KMotRight : Outport  Port=71  VectorParamsAs1DForOutWhenUnconnected=off
  RMotRight : Outport  Port=72  VectorParamsAs1DForOutWhenUnconnected=off
  RMotLeft : Outport  Port=73  VectorParamsAs1DForOutWhenUnconnected=off
  FTarR : Outport  Port=74  VectorParamsAs1DForOutWhenUnconnected=off
  FTarL : Outport  Port=75  VectorParamsAs1DForOutWhenUnconnected=off
  PBCOutDataStorageWrite : Outport  Port=76  VectorParamsAs1DForOutWhenUnconnected=off
  PBCOutDataStorageWrite77 : Outport  Port=77  VectorParamsAs1DForOutWhenUnconnected=off
  PBCInDataStorageRead : Outport  Port=78  VectorParamsAs1DForOutWhenUnconnected=off
  PBCOutDevelopmentMessages : Outport  Port=79  VectorParamsAs1DForOutWhenUnconnected=off
  PBCOutDataStorageWrite80 : Outport  Port=80  VectorParamsAs1DForOutWhenUnconnected=off
  PBCOutDataStorageWrite81 : Outport  Port=81  VectorParamsAs1DForOutWhenUnconnected=off
  PBCInDataStorageRead80 : Outport  Port=82
  PBCInDataStorageRead81 : Outport  Port=83
  PbcSoftwareVersion : Outport  Port=84
  wires:
  Constant4/1 -> [ECUShutDown], Switch/2
  Gain5/1 -> To Workspace5/1, SwOmegaLeft/1  "InternalOmegaL"
  Gain7/1 -> Scope8/2, To Workspace7/1, KMotRight/1, Scope11/2
  Gain6/1 -> KMotLeft/1, Scope14/1, Scope8/1, Scope11/1, To Workspace8/1
  Gain4/1 -> To Workspace6/1, SwOmegaRight/1  "InternalOmegaR"
  Gain10/1 -> To Workspace9/1, RMotLeft/1, Scope6/2, Scope10/2, Scope13/1  "RMotL"
  Gain11/1 -> FTarL/1, To Workspace12/1  "internalFtarL"
  PBCInVariantItem/1 -> Subsystem/1(PBCInVariantItem)
  Gain9/1 -> Scope6/1, To Workspace10/1, RMotRight/1, Scope10/1  "RMotR"
  Gain3/1 -> To Workspace3/1, StrokeLeft/1  "InternalStrokeLeft"
  Gain8/1 -> FTarR/1, To Workspace11/1  "internalFtarR"
  Mux1/1 -> To Workspace20/1
  Pbc_Cyclic/1 -> Terminator1/1
  PBCInMotorDriverStateLeft/1 -> Rate Transition42/1
  Gain2/1 -> To Workspace4/1, StrokeRight/1  "InternalStrokeRight"
  "PBCInDataStorage_Read "/1 -> Switch/3
  Gain1/1 -> To Workspace1/1, FclampLeft/1, Scope15/2  "InternalFestL"
  PBCInDiagRequest/1 -> Data Type Conversion8/1
  HWDriver_MotorVoltageRight_1ms/1 -> Demux5/1
  Mux2/1 -> PbcSoftwareVersion/1
  Gain12/1 -> FclampRight/1, To Workspace2/1, Scope15/1  "InternalFestR"
  PBCInMotorCurrentLeft_1ms/1 -> Scope2/1, Demux2/1
  PBCInDiagOperationMode/1 -> Data Type Conversion7/1
  Mux/1 -> To Workspace21/1
  HWDriver_MotorVoltageLeft_1ms/1 -> Demux4/1
  PBCInMotorCurrentRight_1ms/1 -> Demux3/1
  PBCInFaultRecoveryRequest/1 -> Demux1/1
  PBCinHostSoftwareVersion/1 -> Demux6/1
  Data Type Conversion5/1 -> Switch/1
  PBCInMotorDriverStateRight/1 -> Rate Transition43/1
  OutOfSpec_Init/1 -> Terminator/1
  Constant2/1 -> Mux1/1, Mux/1
  Data Type Conversion1/1 -> Data Type Conversion5/1
  Pbc_Init/1 -> Terminator2/1
  Step/1 -> Data Type Conversion6/1
  S-Function Builder1/1 -> Terminator4/1  "triggerfirstcall"
  Data Type Conversion6/1 -> S-Function Builder1/1
  ApplyReleaseRequest/1 -> S-Function Builder1/2  "ApplyReleaseRequest"
  PBCInDataStorageValid1/1 -> S-Function Builder1/5
  PBCInDataStorageValid2/1 -> S-Function Builder1/6
  PBCInDataStorageRead1/1 -> S-Function Builder1/3
  PBCInDataStorageRead9/1 -> S-Function Builder1/4
  PBCInDataStorageValid3/1 -> S-Function Builder1/7
  Data Type Conversion7/1 -> S-Function Builder1/8
  Data Type Conversion8/1 -> S-Function Builder1/9
  Demux1/40 -> Terminator10/1
  Demux1/39 -> Terminator9/1
  Demux1/38 -> Terminator8/1
  Demux1/37 -> Terminator7/1
  Demux1/1 -> S-Function Builder1/10
  Demux1/2 -> S-Function Builder1/11
  Demux1/3 -> S-Function Builder1/12
  Demux1/4 -> S-Function Builder1/13
  Demux1/5 -> S-Function Builder1/14
  Demux1/6 -> S-Function Builder1/15
  Demux1/7 -> S-Function Builder1/16
  Demux1/8 -> S-Function Builder1/17
  Demux1/9 -> S-Function Builder1/18
  Demux1/10 -> S-Function Builder1/19
  Demux1/11 -> S-Function Builder1/20
  Demux1/12 -> S-Function Builder1/21
  Demux1/13 -> S-Function Builder1/22
  Demux1/14 -> S-Function Builder1/23
  Demux1/15 -> S-Function Builder1/24
  Demux1/16 -> S-Function Builder1/25
  Demux1/17 -> S-Function Builder1/26
  Demux1/18 -> S-Function Builder1/27
  Demux1/19 -> S-Function Builder1/28
  Demux1/20 -> S-Function Builder1/29
  Demux1/21 -> S-Function Builder1/30
  Demux1/22 -> S-Function Builder1/31
  Demux1/23 -> S-Function Builder1/32
  Demux1/24 -> S-Function Builder1/33
  Demux1/25 -> S-Function Builder1/34
  Demux1/26 -> S-Function Builder1/35
  Demux1/27 -> S-Function Builder1/36
  Demux1/28 -> S-Function Builder1/37
  Demux1/29 -> S-Function Builder1/38
  Demux1/30 -> S-Function Builder1/39
  Demux1/31 -> S-Function Builder1/40
  Demux1/32 -> S-Function Builder1/41
  Demux1/33 -> S-Function Builder1/42
  Demux1/35 -> Terminator11/1
  Demux1/36 -> Terminator12/1
  Demux1/34 -> Terminator13/1
  Demux6/2 -> S-Function Builder1/46
  PBCinHostAvailabilityRight/1 -> S-Function Builder1/44
  Demux6/1 -> S-Function Builder1/45
  Demux6/3 -> S-Function Builder1/47
  PBCinHostAvailabilityLeft/1 -> S-Function Builder1/43
  Demux6/4 -> S-Function Builder1/48
  Demux6/5 -> S-Function Builder1/49
  Demux6/6 -> S-Function Builder1/50
  PBCInHpsAvailability/1 -> Scope12/1, S-Function Builder1/51
  PBCInHpsAcknowledge/1 -> Scope25/1, S-Function Builder1/52
  PBCInMasterCylinderPressure/1 -> S-Function Builder1/54
  Demux2/10 -> S-Function Builder1/64
  Demux2/9 -> S-Function Builder1/63
  Demux2/8 -> S-Function Builder1/62
  Demux2/7 -> S-Function Builder1/61
  Demux2/6 -> S-Function Builder1/60
  Demux2/5 -> S-Function Builder1/59
  Demux2/4 -> S-Function Builder1/58
  Demux2/3 -> S-Function Builder1/57
  Demux2/2 -> S-Function Builder1/56
  Demux2/1 -> S-Function Builder1/55
  Demux3/10 -> S-Function Builder1/74
  Demux3/9 -> S-Function Builder1/73
  Demux3/8 -> S-Function Builder1/72
  Demux3/7 -> S-Function Builder1/71
  Demux3/6 -> S-Function Builder1/70
  Demux3/5 -> S-Function Builder1/69
  Demux3/4 -> S-Function Builder1/68
  Demux3/3 -> S-Function Builder1/67
  Demux3/2 -> S-Function Builder1/66
  Demux3/1 -> S-Function Builder1/65
  Rate Transition42/1 -> S-Function Builder1/75
  Rate Transition43/1 -> S-Function Builder1/76
  PBCInMotorDriverSupplyVoltage/1 -> S-Function Builder1/77
  Demux4/10 -> S-Function Builder1/87
  Demux4/9 -> S-Function Builder1/86
  Demux4/8 -> S-Function Builder1/85
  Demux4/7 -> S-Function Builder1/84
  Demux4/6 -> S-Function Builder1/83
  Demux4/5 -> S-Function Builder1/82
  Demux4/4 -> S-Function Builder1/81
  Demux4/3 -> S-Function Builder1/80
  Demux4/2 -> S-Function Builder1/79
  Demux4/1 -> S-Function Builder1/78
  Demux5/10 -> S-Function Builder1/97
  Demux5/9 -> S-Function Builder1/96
  Demux5/8 -> S-Function Builder1/95
  Demux5/7 -> S-Function Builder1/94
  Demux5/6 -> S-Function Builder1/93
  Demux5/5 -> S-Function Builder1/92
  Demux5/4 -> S-Function Builder1/91
  Demux5/3 -> S-Function Builder1/90
  Demux5/2 -> S-Function Builder1/89
  Demux5/1 -> S-Function Builder1/88
  Subsystem/1(Out1) -> S-Function Builder1/102
  PBCInPowerSupplyState/1 -> S-Function Builder1/98
  PBCInRollerBenchActive/1 -> S-Function Builder1/99
  PBCInPbcSleepTime/1 -> S-Function Builder1/100
  PBCInUnexpectedPowerDown/1 -> S-Function Builder1/101
  PBCInWheelPressureFL/1 -> S-Function Builder1/104
  PBCInWheelPressureFR/1 -> S-Function Builder1/105
  PBCInWheelPressureRL/1 -> S-Function Builder1/106
  PBCInWheelPressureRR/1 -> S-Function Builder1/107
  PBCInWheelPressureReliabilityFL/1 -> S-Function Builder1/108
  PBCInWheelPressureReliabilityFR/1 -> S-Function Builder1/109
  PBCInWheelPressureReliabilityRL/1 -> S-Function Builder1/110
  PBCInWheelPressureReliabilityRR/1 -> S-Function Builder1/111
  PBCInWheelPulseFL/1 -> Scope4/1, S-Function Builder1/112
  PBCInWheelPulseFR/1 -> S-Function Builder1/113
  PBCInWheelPulseRL/1 -> S-Function Builder1/114
  PBCInWheelPulseRR/1 -> S-Function Builder1/115
  PBCInWheelSPeedFL/1 -> Scope5/1, S-Function Builder1/116
  PBCInWheelSPeedFR/1 -> S-Function Builder1/117
  PBCInWheelSPeedRL/1 -> S-Function Builder1/118
  PBCInWheelSPeedRR/1 -> S-Function Builder1/119
  PbcInEngineCranking/1 -> S-Function Builder1/120
  PbcInMileage/1 -> S-Function Builder1/121
  PbcInDriveAwayIntentionIndication/1 -> S-Function Builder1/122
  Constant9/1 -> S-Function Builder1/123
  "PBCInDataStorageRead77 "/1 -> S-Function Builder1/124
  Constant/1 -> S-Function Builder1/125, S-Function Builder1/126
  Switch/1 -> PBCInDataStorageRead/1
  Constant1/1 -> PBCInDataStorageRead80/1, PBCInDataStorageRead81/1
  From Workspace/1 -> Data Type Conversion1/1
  S-Function Builder1/14 -> PBCOutDiagRequestStatus/1
  S-Function Builder1/13 -> PBCOutDiagRequestAcknowledge/1
  S-Function Builder1/12 -> PBCOutDiagBrakeTemperatureRight/1
  S-Function Builder1/11 -> PBCOutDiagBrakeTemperatureLeft/1
  S-Function Builder1/10 -> PBCOutDiagActuationCounterRight/1
  S-Function Builder1/9 -> PBCOutDiagActuationCounterLeft/1
  S-Function Builder1/8 -> PBCOutDiagAchievedClampingForceRight/1
  S-Function Builder1/7 -> PBCOutDiagAchievedClampingForceLeft/1
  S-Function Builder1/6 -> PBCOutDevelopmentMessages0/1
  S-Function Builder1/5 -> PBCOutDataStorageWrite9/1
  S-Function Builder1/4 -> PBCOutDataStorageWrite1/1
  S-Function Builder1/3 -> To Workspace19/1, PBCOutActuatorStateRight/1, Scope1/1
  S-Function Builder1/2 -> Scope/1, To Workspace18/1, PBCOutActuatorStateLeft/1
  S-Function Builder1/39 -> Mux4/25, PBCOutFaultStatus_25/1
  S-Function Builder1/38 -> Mux4/24, PBCOutFaultStatus_24/1
  S-Function Builder1/37 -> Mux4/23, PBCOutFaultStatus_23/1
  S-Function Builder1/36 -> Mux4/22, PBCOutFaultStatus_22/1
  S-Function Builder1/35 -> Mux4/21, PBCOutFaultStatus_21/1
  S-Function Builder1/34 -> Mux4/20, PBCOutFaultStatus_20/1
  S-Function Builder1/33 -> Mux4/19, PBCOutFaultStatus_19/1
  S-Function Builder1/32 -> Mux4/18, PBCOutFaultStatus_18/1
  S-Function Builder1/31 -> Mux4/17, PBCOutFaultStatus_17/1
  S-Function Builder1/30 -> Mux4/16, PBCOutFaultStatus_16/1
  S-Function Builder1/29 -> Mux4/15, PBCOutFaultStatus_15/1
  S-Function Builder1/28 -> Mux4/14, PBCOutFaultStatus_14/1
  S-Function Builder1/27 -> Mux4/13, PBCOutFaultStatus_13/1
  S-Function Builder1/26 -> Mux4/12, PBCOutFaultStatus_12/1
  S-Function Builder1/25 -> Mux4/11, PBCOutFaultStatus_11/1
  S-Function Builder1/24 -> Mux4/10, PBCOutFaultStatus_10/1
  S-Function Builder1/23 -> Mux4/9, PBCOutFaultStatus_09/1
  S-Function Builder1/22 -> Mux4/8, PBCOutFaultStatus_08/1
  S-Function Builder1/21 -> Mux4/7, PBCOutFaultStatus_07/1
  S-Function Builder1/20 -> Mux4/6, PBCOutFaultStatus_06/1
  S-Function Builder1/19 -> Mux4/5, PBCOutFaultStatus_05/1
  S-Function Builder1/18 -> Mux4/4, PBCOutFaultStatus_04/1
  S-Function Builder1/17 -> Mux4/3, PBCOutFaultStatus_03/1
  S-Function Builder1/16 -> Mux4/2, PBCOutFaultStatus_02/1
  S-Function Builder1/15 -> Mux4/1, PBCOutFaultStatus_01/1
  S-Function Builder1/54 -> Scope7/1, PBCOutHpsPressure/1
  S-Function Builder1/53 -> Mux4/39, PBCOutFaultStatus_39/1
  S-Function Builder1/52 -> Mux4/38, PBCOutFaultStatus_38/1
  S-Function Builder1/51 -> Mux4/37, PBCOutFaultStatus_37/1
  S-Function Builder1/50 -> Mux4/36, PBCOutFaultStatus_36/1
  S-Function Builder1/49 -> Mux4/35, PBCOutFaultStatus_35/1
  S-Function Builder1/48 -> Mux4/34, PBCOutFaultStatus_34/1
  S-Function Builder1/47 -> Mux4/33, PBCOutFaultStatus_33/1
  S-Function Builder1/46 -> Mux4/32, PBCOutFaultStatus_32/1
  S-Function Builder1/45 -> Mux4/31, PBCOutFaultStatus_31/1
  S-Function Builder1/44 -> Mux4/30, PBCOutFaultStatus_30/1
  S-Function Builder1/43 -> Mux4/29, PBCOutFaultStatus_29/1
  S-Function Builder1/42 -> Mux4/28, PBCOutFaultStatus_28/1
  S-Function Builder1/41 -> PBCOutFaultStatus_27/1, Mux4/27
  S-Function Builder1/40 -> Mux4/26, PBCOutFaultStatus_26/1
  S-Function Builder1/58 -> PBCOutOfSpecMsg/1
  S-Function Builder1/57 -> Scope22/1, PBCOutMotorCommandRight/1
  S-Function Builder1/56 -> Scope27/1, PBCOutMotorCommandLeft/1
  S-Function Builder1/55 -> Scope3/1, PBCOutHpsRequest/1
  S-Function Builder1/59 -> Mux2/1
  S-Function Builder1/60 -> Mux2/2
  S-Function Builder1/61 -> Mux2/3
  S-Function Builder1/62 -> Mux2/4
  S-Function Builder1/63 -> Mux2/5
  S-Function Builder1/64 -> Mux2/6
  S-Function Builder1/65 -> PBCOutEcuPowerLatchRequest/1
  S-Function Builder1/66 -> Gain12/1
  S-Function Builder1/67 -> Gain1/1
  S-Function Builder1/68 -> Gain2/1
  S-Function Builder1/69 -> Gain3/1
  S-Function Builder1/70 -> Gain4/1
  S-Function Builder1/71 -> Gain5/1
  S-Function Builder1/72 -> Gain7/1
  S-Function Builder1/73 -> Gain6/1
  S-Function Builder1/74 -> Gain9/1
  S-Function Builder1/75 -> Gain10/1
  S-Function Builder1/76 -> Gain8/1
  S-Function Builder1/77 -> Gain11/1
  S-Function Builder1/78 -> To Workspace13/1
  S-Function Builder1/79 -> To Workspace14/1
  S-Function Builder1/80 -> PbcOutPadAdjustmentRequest/1
  S-Function Builder1/81 -> PbcOutParkSupportRequest/1
  S-Function Builder1/82 -> "PbcOutDataStorageRequest "/1
  S-Function Builder1/83 -> triggerrecal/1
  PBCInLongAcceleration/1 -> Scope28/1, S-Function Builder1/53
  PBCInVehicleAmbientTemperature/1 -> S-Function Builder1/103
  Mux4/1 -> To Workspace/1
